simulink model "State_Machine"  (R2024a)
settings: Solver=FixedStepDiscrete  StartTime=0.0  StopTime=10000  RelTol=1e-3
PreLoadFcn:
  | clearEnums;
model workspace (MAT data in the model file):
  Active_Scenario_Index = 1
  BattTempInit = 25
  Battery.SOC_LUT = [0.01 0.02 0.03 0.04 0.05 0.06 0.07 0.08 0.09 0.1 0.11 0.12 0.13 0.14 0.15 0.16 0.17 0.18 0.19 0.2 0.21 0.22 0.23 0.24 0.25 0.26 0.27 0.28 0.29 0.3 0.31 0.32 0.33 0.34 0.35 0.36 0.37 0.38 0.39 0.4 0.41 0.42 0.43 0.44 0.45 0.46 0.47 0.48 0.49 0.5 0.51 0.52 0.53 0.54 0.55 0.56 0.57 0.58 0.59 0.6 0.61 0.62 0.63 0.64 0.65 0.66 0.67 0.68 0.69 0.7 0.71 0.72 0.73 0.74 0.75 0.76 0.77 0.78 0.79 0.8 0.81 0.82 0.83 0.84 0.85 0.86 0.87 0.88 0.89 0.9 0.91 0.92 0.93 0.94 0.95 0.96 0.97 0.98 0.99 1]
  Battery.Temperature_LUT = [-10 0 25 40]
  Battery.Capacity_LUT = [4.04528301887 4.19622641509 4.8 4.73962264151]
  Battery.Em_LUT = [2.67308083891 2.74411674384 2.80408613071 2.86247711994 2.90851059763 2.94904306488 2.9829846776 3.01467102589 3.04031502638 3.06256828113 3.08180972392 3.09994219643 ... (400 elements, 100x4)]
  Battery.R0_LUT = [0.0569026752707 0.0575506938969 0.0576730924021 0.0575627404981 0.0573787336615 0.0571931123197 0.0568199985482 0.056411926464 0.0561974340667 0.0560805640861 0.0557640899305 0.055275807865 ... (400 elements, 100x4)]
  Battery.R1_LUT = [0.0035 0.0035 0.0035 0.0035 0.0035 0.0035 0.0035 0.0035 0.0035 0.0035 0.0035 0.0035 ... (400 elements, 100x4)]
  Battery.C1_LUT = [5000 5000 5000 5000 5000 5000 5000 5000 5000 5000 5000 5000 ... (400 elements, 100x4)]
  Battery.Mass = 0.047
  Battery.ThermalMass = 44
  Battery.R_bleed = 20
  Battery.h_conv = 5
  Battery.cell_area = 0.0037
  Battery.TempInit = 25
  Battery.SOCInit = 0.75
  Battery.Model = 'panasonic ncr18650bd'
  Battery.DischargeCycle_LUT = [1 5 9 13 17 21 25 29 33 37 41 45 49 53 57 61 65 69 73 77 81 85 89 93 97 101 105 109 113 117 121 125 129 133 137 141 145 149 153 157 161 165 169 173 177 181 185 189 193 197 201 205 209 213 217 221 225 229 233 237 241 245 249 253 257 261 265 269 273 277 281 285 289 293 297 301 305 309 313 317]
  Battery.deltaEm_LUT = [0 -0.363115641304 -0.600096647258 -0.689070000839 -0.76773380251 -0.846397604181 -0.926368385458 -0.992711297521 -1.05704974111 -1.12227693902 -1.19018070587 -1.25808447272 -1.31699459748 -1.35876443799 -1.40168267642 -1.44460091485 -1.48751915327 -1.5304373917 -1.57335563013 -1.62198241593 -1.67232184498 -1.71858340023 -1.76179802551 -1.8050126508 -1.84822727608 -1.8917937136 -1.93575272784 -1.97971174208 -2.02367075632 -2.06762977056 -2.11171979109 -2.15588700406 -2.19980020032 -2.24365853098 -2.28751686164 -2.33137519231 -2.37523352297 -2.41909185363 -2.45982559031 -2.49599372373 -2.53216185715 -2.56832999058 -2.604498124 -2.64066625743 -2.67683439085 -2.71300252428 -2.7491706577 -2.78367585394 -2.81632179346 -2.8483348579 -2.88034792233 -2.91236098677 -2.94437405121 -2.97638711564 -3.00840018008 -3.04041324451 -3.07260346059 -3.10359008254 -3.13082308991 -3.15805609728 -3.18528910464 -3.21252211201 -3.23975511938 -3.26698812675 -3.29422113412 -3.32122400938 -3.3463475604 -3.37152613073 -3.39670470105 -3.42188327138 -3.4470618417 -3.47224041203 -3.49938358795 -3.52900276724 -3.55862194653 -3.58824112582 -3.6178603051 -3.64748858268 -3.67711690909 -3.70674523549]
  Battery.deltaCapacity_LUT = [0 -0.860019120059 -1.71332421702 -2.0819400264 -2.45055583577 -2.81917164515 -3.18778745452 -3.48884924257 -3.7808148236 -4.07278040463 -4.36474598566 -4.6567115667 -4.91000721732 -5.08494410056 -5.2598809838 -5.43481786703 -5.60975475027 -5.78469163351 -5.95962851674 -6.13456539998 -6.30950228322 -6.47026795816 -6.62044510558 -6.77062225299 -6.92079940041 -7.07097654783 -7.22115369524 -7.37133084266 -7.52150799007 -7.67168513749 -7.82230984162 -7.97319825819 -8.12408667477 -8.27497509134 -8.42586350792 -8.57675192449 -8.72764034107 -8.87852875764 -9.01789522921 -9.13717923376 -9.25646323831 -9.37574724285 -9.4950312474 -9.61431525195 -9.73359925649 -9.85288326104 -9.97216726558 -10.0914512701 -10.2059878191 -10.3183039593 -10.4306200996 -10.5429362398 -10.65525238 -10.7675685203 -10.8798846605 -10.9922008008 -11.104516941 -11.2125891929 -11.3075699376 -11.4025506823 -11.4975314271 -11.5925121718 -11.6874929166 -11.7824736613 -11.877454406 -11.9716325175 -12.0588579537 -12.1460833899 -12.2333088261 -12.3205342623 -12.4077596986 -12.4949851348 -12.5890165008 -12.6916254178 -12.7942343349 -12.8968432519 -12.999452169 -13.102061086 -13.2046700031 -13.3072789201]
  Battery.cond_thickness = 0.001
  Battery.thermal_conductivity = 205
  CV_Gain = 0.20000000298
  CellType = 1
  HighTempDchrgCurrentLim = Simulink.Signal
  HighTempDchrgCurrentLim.DataType = 'single'
  HighTempDchrgCurrentLim.Dimensions = -1
  HighTempDchrgCurrentLim.DimensionsMode = 'auto'
  HighTempDchrgCurrentLim.Complexity = 'auto'
  HighTempDchrgCurrentLim.SampleTime = -1
  HighTempDchrgCurrentLim.SamplingMode = 'auto'
  HighTempLimit = 50
  I_cc = 30
  LowTempDchrgCurrentLim = Simulink.Signal
  LowTempDchrgCurrentLim.DataType = 'single'
  LowTempDchrgCurrentLim.Dimensions = -1
  LowTempDchrgCurrentLim.DimensionsMode = 'auto'
  LowTempDchrgCurrentLim.Complexity = 'auto'
  LowTempDchrgCurrentLim.SampleTime = -1
  LowTempDchrgCurrentLim.SamplingMode = 'auto'
  LowTempLimit = 5
  MaxCellVoltThrsld = 4.19999980927
  MaxChrgCurrLim = Simulink.Parameter
  MaxChrgCurrLim.Value = 6.36000013351
  MaxChrgCurrLim.Complexity = 'real'
  MaxChrgCurrLim.Dimensions = [1 1]
  MaxChrgCurrLim.DataType = 'single'
  MaxDchrgCurrLim = Simulink.Parameter
  MaxDchrgCurrLim.Value = -20
  MaxDchrgCurrLim.Complexity = 'real'
  MaxDchrgCurrLim.Dimensions = [1 1]
  MaxDchrgCurrLim.DataType = 'single'
  MinCellVoltDchrgCurrentLim = Simulink.Signal
  MinCellVoltDchrgCurrentLim.DataType = 'single'
  MinCellVoltDchrgCurrentLim.Dimensions = -1
  MinCellVoltDchrgCurrentLim.DimensionsMode = 'auto'
  MinCellVoltDchrgCurrentLim.Complexity = 'auto'
  MinCellVoltDchrgCurrentLim.SampleTime = -1
  MinCellVoltDchrgCurrentLim.SamplingMode = 'auto'
  MinCellVoltDchrgCurrentLimTable = Simulink.LookupTable
  MinCellVoltDchrgCurrentLimTable.Table = Simulink.lookuptable.Table
  MinCellVoltDchrgCurrentLimTable.Table.Value = [0 0.5 1]
  MinCellVoltDchrgCurrentLimTable.Table.Dimensions = [1 3]
  MinCellVoltDchrgCurrentLimTable.Table.DataType = 'single'
  MinCellVoltDchrgCurrentLimTable.Table.FieldName = 'DischargeCurrentRate'
  MinCellVoltDchrgCurrentLimTable.Table.Description = 'Discharge Current Rate Based On Mim Cell Voltage'
  MinCellVoltDchrgCurrentLimTable.Breakpoints = Simulink.lookuptable.Breakpoint
  MinCellVoltDchrgCurrentLimTable.Breakpoints.Value = [2.5; 2.75; 3]
  MinCellVoltDchrgCurrentLimTable.Breakpoints.TunableSizeName = 'N1'
  MinCellVoltDchrgCurrentLimTable.Breakpoints.Dimensions = [3 1]
  MinCellVoltDchrgCurrentLimTable.Breakpoints.DataType = 'single'
  MinCellVoltDchrgCurrentLimTable.Breakpoints.Unit = 'V'
  MinCellVoltDchrgCurrentLimTable.Breakpoints.FieldName = 'MinCellVoltage'
  MinCellVoltDchrgCurrentLimTable.Breakpoints.Description = 'Minimum Cell Voltage'
  MinCellVoltDchrgCurrentLimTable.AllowMultipleInstancesOfTypeToHaveDifferentTableBreakpointSizes = 0
  MinCellVoltDchrgCurrentLimTable.SupportTunableSize = 0
  MinCellVoltDchrgCurrentLimTable.StructTypeInfo = Simulink.lookuptable.StructTypeInfo
  MinCellVoltDchrgCurrentLimTable.StructTypeInfo.Name = 'MinCellVoltDchrgCurrentLimTable'
  MinCellVoltDchrgCurrentLimTable.StructTypeInfo.DataScope = 'Auto'
  Np_Module = 31
  Ns_Module = 24
  NumModules = 4
  OverCellVoltageLimit = 4.19999980927
  Sig = Simulink.Signal
  Sig.DataType = 'auto'
  Sig.Dimensions = -1
  Sig.DimensionsMode = 'auto'
  Sig.Complexity = 'auto'
  Sig.SampleTime = -1
  Sig.SamplingMode = 'auto'
  SnsrFltThld = 0.252
  TestCase = 1
  UnderCellVoltageLimit = 2.5
  contactorTime = 200
  currentFactor = 10
  noCurrent = 0
  timeoutContactor = 1
  timeoutCurrent = 1
  ts = 0.1
  vRatio = 0.949999988079
  voltThreshold = 4.09999990463
settings Model: DataDictionary=DD_State_Machine.sldd  ModifiedByFormat=The MathWorks, Inc.  ExtModeTrigDuration=5  Creator=The MathWorks, Inc.  LastModifiedBy=The MathWorks, Inc.
settings SolverCC: AlgebraicLoopSolver=TrustRegion  PositivePriorityOrder=on  AutoInsertRateTranBlk=on  MaxZcPerStep=1
settings DataIOCC: ExternalInput=Battery  SaveOutput=off  SaveTime=off  SignalLoggingName=logsOut
settings OptimizationCC: BlockReduction=off  DefaultParameterBehavior=Inlined  UseFloatMulNetSlope=on  DefaultUnderspecifiedDataType=single  OptimizeBlockIOStorage=off  EnhancedBackFolding=on  PassReuseOutputArgsThreshold=0  ZeroExternalMemoryAtStartup=off  ZeroInternalMemoryAtStartup=off  EfficientFloat2IntCast=on  MaxStackSize=64  OptimizeBlockOrder=speed  DifferentSizesBufferReuse=on
settings DebuggingCC: SignalInfNanChecking=error  SaveWithParameterizedLinksMsg=none  CheckExecutionContextPreStartOutputMsg=on  IntegerOverflowMsg=error  ParameterPrecisionLossMsg=none  ParameterTunabilityLossMsg=error  UnconnectedInputMsg=warning  UnconnectedOutputMsg=warning  UnconnectedLineMsg=warning  AssertControl=DisableAll  PregeneratedLibrarySubsystemCodeDiagnostic=none  SFUnexpectedBacktrackingDiag=warning  SFNoUnconditionalDefaultTransitionDiag=warning  SFExecutionAtInitializationDiag=none  ArithmeticOperatorsInVariantConditions=warning
settings HardwareCC: ProdBitPerLong=64  ProdLongLongMode=on  ProdHWDeviceType=Intel->x86-64 (Linux 64)
settings ModelReferenceCC: EnableRefExpFcnMdlSchedulingChecks=on  ModelReferenceNumInstancesAllowed=Single  PropagateSignalLabelsOutOfModel=off
settings SFSimCC: SimUseLocalCustomCode=off  MATLABDynamicMemAlloc=off  CustomCodeUndefinedFunction=UseInterfaceOnly
settings RTWCC: GenerateReport=on  RTWUseLocalCustomCode=off  BuildConfiguration=Faster Runs  TargetLang=C++  GPUComputeCapability=3.5  DLArmComputeVersion=19.05
settings CodeAppCC: ForceParamTrailComments=on  MaxIdLength=51  OperatorAnnotations=on  MangleLength=4
settings GRTTargetCC: TargetLangStandard=C++03 (ISO)  CodeInterfacePackaging=C++ class
settings ConfigComp: CovMetricSettings=dcw  CovSaveCumulativeToWorkspaceVar=on  CovSaveSingleToWorkspaceVar=on  CovExternalEMLEnable=off  CovSFcnEnable=off  DVMode=DesignErrorDetection  DVMaxProcessTime=7000  DVTestSuiteOptimization=Auto  DVDetectDeadLogic=on  DVDetectIntegerOverflow=off  DVRebuildModelRepresentation=Always

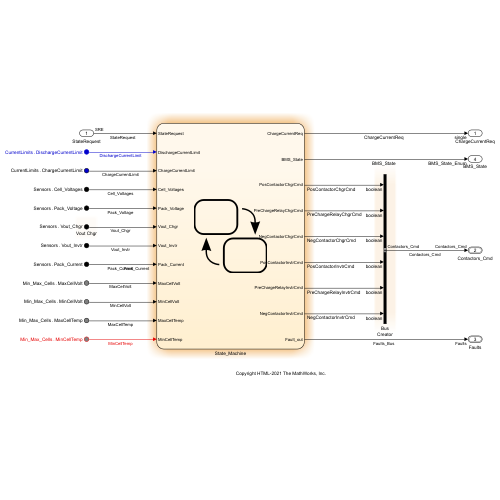
[thumbnail: Simulink's stored preview of the top-level diagram]
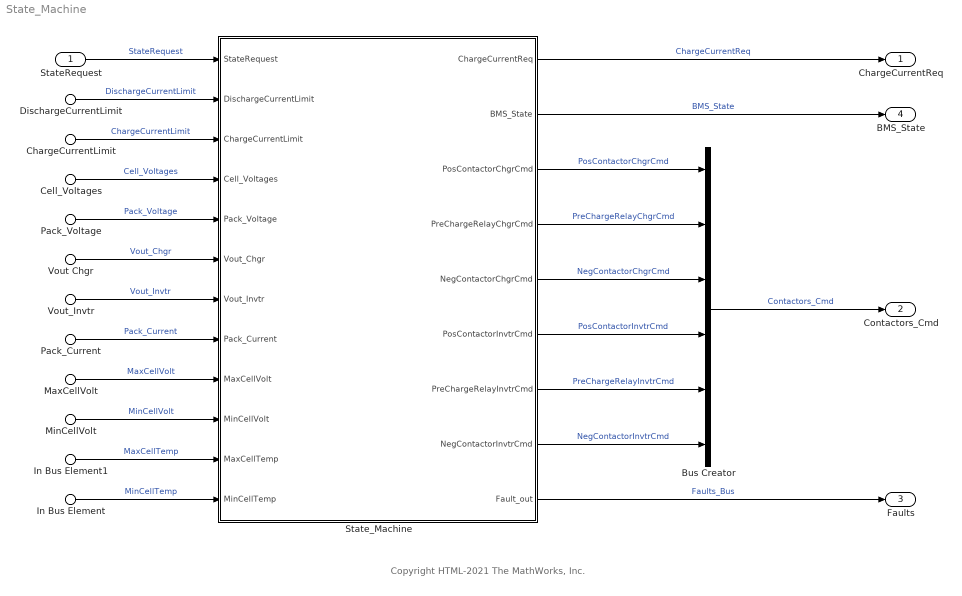
== system State_Machine ==
  note: Copyright HTML-2021 The MathWorks, Inc.
  StateRequest : Inport  OutDataTypeStr=Enum: SRE  PortDimensions=1  SampleTime=[0.10000000000000001,0]
  Cell_Voltages : Inport  Port=2  PortName=Sensors  Element=Cell_Voltages
  Pack_Voltage : Inport  Port=2  PortName=Sensors  Element=Pack_Voltage
  Pack_Current : Inport  Port=2  PortName=Sensors  Element=Pack_Current
  Vout Chgr : Inport  Port=2  PortName=Sensors  Element=Vout_Chgr
  Vout_Invtr : Inport  Port=2  PortName=Sensors  Element=Vout_Invtr
  DischargeCurrentLimit : Inport  Port=3  PortName=CurrentLimits  Element=DischargeCurrentLimit
  ChargeCurrentLimit : Inport  Port=3  PortName=CurrentLimits  Element=ChargeCurrentLimit
  MinCellVolt : Inport  Port=4  PortName=Min_Max_Cells  Element=MinCellVolt
  MaxCellVolt : Inport  Port=4  PortName=Min_Max_Cells  Element=MaxCellVolt
  In Bus Element : Inport  Port=4  PortName=Min_Max_Cells  Element=MinCellTemp
  In Bus Element1 : Inport  Port=4  PortName=Min_Max_Cells  Element=MaxCellTemp
  Bus Creator : BusCreator  Inputs=6  OutDataTypeStr=Bus: Contactors_Cmd  NonVirtualBus=on
      settings: InheritFromInputs=off
  State_Machine : Stateflow chart  TreatAsAtomicUnit=on  VariantControl=(default)
  ChargeCurrentReq : Outport  OutMin=-100  OutMax=100  OutDataTypeStr=single  PortDimensions=1  SampleTime=[0.10000000000000001,0]  VectorParamsAs1DForOutWhenUnconnected=off
  Contactors_Cmd : Outport  Port=2  OutDataTypeStr=Bus: Contactors_Cmd  BusOutputAsStruct=on
  Faults : Outport  Port=3  OutDataTypeStr=Bus: Faults  VectorParamsAs1DForOutWhenUnconnected=off  BusOutputAsStruct=on
  BMS_State : Outport  Port=4  OutDataTypeStr=Enum: BMS_State_Enum  PortDimensions=1  SampleTime=[0.10000000000000001,0]  VectorParamsAs1DForOutWhenUnconnected=off
  wires:
  State_Machine/2(BMS_State) -> BMS_State/1  "BMS_State"
  State_Machine/1(ChargeCurrentReq) -> ChargeCurrentReq/1  "ChargeCurrentReq"
  State_Machine/3(PosContactorChgrCmd) -> Bus Creator/1  "PosContactorChgrCmd"
  State_Machine/4(PreChargeRelayChgrCmd) -> Bus Creator/2  "PreChargeRelayChgrCmd"
  State_Machine/5(NegContactorChgrCmd) -> Bus Creator/3  "NegContactorChgrCmd"
  State_Machine/6(PosContactorInvtrCmd) -> Bus Creator/4  "PosContactorInvtrCmd"
  State_Machine/7(PreChargeRelayInvtrCmd) -> Bus Creator/5  "PreChargeRelayInvtrCmd"
  State_Machine/8(NegContactorInvtrCmd) -> Bus Creator/6  "NegContactorInvtrCmd"
  State_Machine/9(Fault_out) -> Faults/1  "Faults_Bus"
  DischargeCurrentLimit/1 -> State_Machine/2(DischargeCurrentLimit)  "DischargeCurrentLimit"
  ChargeCurrentLimit/1 -> State_Machine/3(ChargeCurrentLimit)  "ChargeCurrentLimit"
  Cell_Voltages/1 -> State_Machine/4(Cell_Voltages)  "Cell_Voltages"
  MinCellVolt/1 -> State_Machine/10(MinCellVolt)  "MinCellVolt"
  MaxCellVolt/1 -> State_Machine/9(MaxCellVolt)  "MaxCellVolt"
  StateRequest/1 -> State_Machine/1(StateRequest)  "StateRequest"
  Pack_Current/1 -> State_Machine/8(Pack_Current)  "Pack_Current"
  Vout_Invtr/1 -> State_Machine/7(Vout_Invtr)  "Vout_Invtr"
  Vout Chgr/1 -> State_Machine/6(Vout_Chgr)  "Vout_Chgr"
  Pack_Voltage/1 -> State_Machine/5(Pack_Voltage)  "Pack_Voltage"
  Bus Creator/1 -> Contactors_Cmd/1  "Contactors_Cmd"
  In Bus Element1/1 -> State_Machine/11(MaxCellTemp)  "MaxCellTemp"
  In Bus Element/1 -> State_Machine/12(MinCellTemp)  "MinCellTemp"

== stateflow chart State_Machine/State_Machine ==
  state Fault Monitoring [group]
    state MonitorCurrLim [parallel]
      settings: executionOrder=1
      state Wait
      state NoCurrLimFault
      state OverCurrentFault
        en:
        FaultPresent = true;
        Fault_out.OverCurrent=true;
      (default) -> NoCurrLimFault : {FaultPresent = false;
          | Fault_out.OverCurrent=false;}
      NoCurrLimFault -> Wait : [(Pack_Current < DischargeCurrentLimit) || ...
          | (Pack_Current > ChargeCurrentLimit)]
      Wait -> NoCurrLimFault [order 2] : [(Pack_Current >= DischargeCurrentLimit) && ...
          | (Pack_Current <= ChargeCurrentLimit)]
      Wait -> OverCurrentFault [order 1] : [after(timeoutCurrent,sec)]
    state MonitorCellVoltage [parallel]
      settings: executionOrder=2
      state OverVoltageFault
        en:
        FaultPresent = true;
        Fault_out.OverVolt = true;
      state NoCellVoltFault
        en,du:
        Delta = abs(Pack_Voltage - sum(Cell_Voltages));
      state SensorFaut
        en:
        FaultPresent = true;
        Fault_out.VoltSensor = true;
      state UnderVoltageFault
        en:
        FaultPresent = true;
        Fault_out.UnderVolt = true;
      (default) -> NoCellVoltFault : {FaultPresent = false;
          | Fault_out.OverVolt = false;
          | Fault_out.UnderVolt = false;
          | Fault_out.VoltSensor = false;
          | }
      NoCellVoltFault -> OverVoltageFault [order 1] : [MaxCellVolt >= ...
          | OverCellVoltageLimit]
      NoCellVoltFault -> SensorFaut [order 2] : [Delta >=...
          |  single(SnsrFltThld)]
      NoCellVoltFault -> UnderVoltageFault [order 3] : [MinCellVolt <=...
          |  UnderCellVoltageLimit]
    state MonitorCellTemp [parallel]
      settings: executionOrder=3
      state HighTemperatureFault
        en:
        FaultPresent = true;
        Fault_out.HighTemp = true;
      state NoCellTempFault
      state LowTemperatureFault
        en:
        FaultPresent = true;
        Fault_out.LowTemp = true;
      (default) -> NoCellTempFault : {FaultPresent = false;
          | Fault_out.HighTemp = false;
          | Fault_out.LowTemp = false;}
      NoCellTempFault -> HighTemperatureFault [order 1] : [MaxCellTemp >= HighTempLimit]
      NoCellTempFault -> LowTemperatureFault [order 2] : [MinCellTemp <= LowTempLimit]
  state MainStateMachine [parallel]
    settings: executionOrder=1
    state Charging
      en:
      BMS_State = BMS_State_Enum.BMS_Charging;
      state Init_Mode
        en:
        ChargeModeReq = Charge_Mode_Enum.Init_Mode;
        ChargeCurrentReq = noCurrent;
      state CC_Mode
        en:
        ChargeModeReq = Charge_Mode_Enum.CC_Mode;
        du:
        ChargeCurrentReq = min(I_cc,ChargeCurrentLimit);
      state CV_Mode
        en:
        ChargeModeReq = Charge_Mode_Enum.CV_Mode;
        du:
        ChargeCurrentReq = ChargeCurrentReq - CV_Gain*(MaxCellVolt - MaxCellVoltThrsld);
        ChargeCurrentReq = min(ChargeCurrentReq, ChargeCurrentLimit);
      (default) -> Init_Mode
      CV_Mode -> Init_Mode : [StateRequest ~= SRE.Charging || ...
          | ChargeCurrentReq <= (I_cc/currentFactor)]
      CC_Mode -> Init_Mode [order 1] : [StateRequest ~= SRE.Charging]
      Init_Mode -> CC_Mode : [StateRequest == SRE.Charging && ...
          | MaxCellVolt < voltThreshold]
      CC_Mode -> CV_Mode [order 2] : [MaxCellVolt>=...
          | MaxCellVoltThrsld]
    state Standby
      en:
      BMS_State = ...
      BMS_State_Enum.BMS_Standby;
    state Driving
      en:
      BMS_State = ...
      BMS_State_Enum.BMS_Driving;
    state Fault
      en,du:
      BMS_State = BMS_State_Enum.BMS_Fault;
    (default) -> Standby
    Standby -> (junction 577) [order 1] : [FaultPresent]
    Standby -> Charging [order 2] : [StateRequest ==SRE.Charging...
        | && ChrgCntctState == Contact.Close]
    (junction 577) -> (junction 580)
    Charging -> Standby [order 3] : [StateRequest ~=SRE.Charging...
        |  && ChrgCntctState == Contact.Init]
    Standby -> Driving [order 3] : [StateRequest == SRE.Driving && ...
        | InvtrCntctState == Contact.Close]
    Driving -> Standby [order 3] : [StateRequest ~= SRE.Driving && ...
        | InvtrCntctState == Contact.Init]
    Driving -> Charging [order 2] : [StateRequest == SRE.Charging && ...
        | ChrgCntctState == Contact.Close]
    Charging -> Driving [order 2] : [StateRequest == SRE.Driving && ...
        | InvtrCntctState == Contact.Close]
    Driving -> Fault [order 1] : [FaultPresent]
    Charging -> Fault [order 1] : [FaultPresent]{ChargeCurrentReq = single(0);}
    (junction 580) -> Fault
  state ChargerContactorState [parallel]
    settings: executionOrder=2
    state OpenChgrContactors
      state ClosePreChrgRly
        PreChargeRelayChgrCmd = true;
      state OpenPosCntct
        PosContactorChgrCmd = false;
      state OpenPreChrgRly
        PreChargeRelayChgrCmd = false;
      state OpenNegCntct
        NegContactorChgrCmd = false;
        ChrgCntctState = Contact.Open;
        PreChrgFault = false;
        Fault_out.Charger = false;
      (default) -> ChargerContactorState.OpenChgrContactors.ClosePreChrgRly : {ChrgCntctState = Contact.Init;}
      ChargerContactorState.OpenChgrContactors.ClosePreChrgRly -> ChargerContactorState.OpenChgrContactors.OpenPosCntct : after(contactorTime,msec) % Check for low current
      ChargerContactorState.OpenChgrContactors.OpenPosCntct -> ChargerContactorState.OpenChgrContactors.OpenPreChrgRly : after(contactorTime,msec)
      ChargerContactorState.OpenChgrContactors.OpenPreChrgRly -> ChargerContactorState.OpenChgrContactors.OpenNegCntct : after(contactorTime,msec)
    state CloseChgrContactors
      state CloseNegCntct
        NegContactorChgrCmd = true;
      state ClosePreChrgRly
        PreChargeRelayChgrCmd = true;
      state ClosePosCntct
        PosContactorChgrCmd = true;
      state OpenPreChrgRly
        PreChargeRelayChgrCmd = false;
        ChrgCntctState = Contact.Close;
      state PreChrgFlt
        PreChrgFault = true;
        Fault_out.Charger = true;
      (default) -> ChargerContactorState.CloseChgrContactors.CloseNegCntct : {ChrgCntctState = Contact.Init;}
      ChargerContactorState.CloseChgrContactors.CloseNegCntct -> ChargerContactorState.CloseChgrContactors.ClosePreChrgRly : after(contactorTime,msec)
      ChargerContactorState.CloseChgrContactors.ClosePreChrgRly -> (junction 564) [order 2]
      (junction 564) -> (junction 566) : after(timeoutContactor,sec)
          | % Check timeout
      ChargerContactorState.CloseChgrContactors.ClosePreChrgRly -> ChargerContactorState.CloseChgrContactors.ClosePosCntct [order 1] : [Vout_Chgr/Pack_Voltage >=vRatio]
      ChargerContactorState.CloseChgrContactors.ClosePosCntct -> ChargerContactorState.CloseChgrContactors.OpenPreChrgRly : after(contactorTime,msec)
      (junction 566) -> ChargerContactorState.CloseChgrContactors.PreChrgFlt
    (default) -> OpenChgrContactors : {ChrgCntctState = Contact.Init;
        | PreChrgFault = false;
        | Fault_out.Charger = false;}
    CloseChgrContactors -> OpenChgrContactors : [StateRequest ~= SRE.Charging || ...
        | FaultPresent]
    OpenChgrContactors -> CloseChgrContactors : [StateRequest == SRE.Charging && ...
        | InvtrCntctState == Contact.Open && ...
        | ~FaultPresent]
  state InverterContactorState [parallel]
    settings: executionOrder=3
    state CloseInvtrContactors
      state CloseNegCntct
        NegContactorInvtrCmd = true;
      state ClosePreChrgRly
        PreChargeRelayInvtrCmd = true;
      state ClosePosCntct
        PosContactorInvtrCmd = true;
      state OpenPreChrgRly
        PreChargeRelayInvtrCmd = false;
        InvtrCntctState = Contact.Close;
      state PreChrgFlt
        PreChrgFault = true;
        Fault_out.Inverter = true;
      (default) -> InverterContactorState.CloseInvtrContactors.CloseNegCntct : {InvtrCntctState = Contact.Init;}
      InverterContactorState.CloseInvtrContactors.CloseNegCntct -> InverterContactorState.CloseInvtrContactors.ClosePreChrgRly : after(contactorTime,msec)
      InverterContactorState.CloseInvtrContactors.ClosePreChrgRly -> (junction 569) [order 2]
      (junction 569) -> (junction 570) : after(timeoutContactor,sec)
          | % Check timeout
      InverterContactorState.CloseInvtrContactors.ClosePreChrgRly -> InverterContactorState.CloseInvtrContactors.ClosePosCntct [order 1] : [Vout_Invtr/Pack_Voltage >=vRatio]
      InverterContactorState.CloseInvtrContactors.ClosePosCntct -> InverterContactorState.CloseInvtrContactors.OpenPreChrgRly : after(contactorTime,msec)
      (junction 570) -> InverterContactorState.CloseInvtrContactors.PreChrgFlt
    state OpenInvtrContactors
      state ClosePreChrgRly
        PreChargeRelayInvtrCmd = true;
      state OpenPosCntct
        PosContactorInvtrCmd = false;
      state OpenPreChrgRly
        PreChargeRelayInvtrCmd = false;
      state OpenNegCntct
        NegContactorInvtrCmd = false;
        InvtrCntctState = Contact.Open;
        PreChrgFault = false;
        Fault_out.Inverter = false;
      (default) -> InverterContactorState.OpenInvtrContactors.ClosePreChrgRly : {InvtrCntctState = Contact.Init;}
      InverterContactorState.OpenInvtrContactors.ClosePreChrgRly -> InverterContactorState.OpenInvtrContactors.OpenPosCntct : after(contactorTime,msec) % Check for low current
      InverterContactorState.OpenInvtrContactors.OpenPosCntct -> InverterContactorState.OpenInvtrContactors.OpenPreChrgRly : after(contactorTime,msec)
      InverterContactorState.OpenInvtrContactors.OpenPreChrgRly -> InverterContactorState.OpenInvtrContactors.OpenNegCntct : after(contactorTime,msec)
    (default) -> OpenInvtrContactors : {InvtrCntctState =Contact.Init;
        | PreChrgFault = false;
        | Fault_out.Inverter = false;}
    CloseInvtrContactors -> OpenInvtrContactors : [StateRequest ~= SRE.Driving || ...
        | FaultPresent]
    OpenInvtrContactors -> CloseInvtrContactors : [StateRequest == SRE.Driving && ...
        | ChrgCntctState == Contact.Open && ...
        | ~FaultPresent]
  data: StateRequest input Enum: SRE; DischargeCurrentLimit input single; ChargeCurrentLimit input single; Cell_Voltages input single; Pack_Voltage input single; Vout_Chgr input single; Vout_Invtr input single; Pack_Current input single; ChargeCurrentReq output; I_cc parameter; MaxCellVolt input single; BMS_State output Enum: BMS_State_Enum =BMS_State_Enum.BMS_Standby; PosContactorChgrCmd output boolean; PreChargeRelayChgrCmd output; NegContactorChgrCmd output; PosContactorInvtrCmd output; PreChargeRelayInvtrCmd output; NegContactorInvtrCmd output; ChrgCntctState local Enum: Contact; InvtrCntctState local Enum: Contact; PreChrgFault local; MaxCellVoltThrsld parameter; FaultPresent local; MinCellVolt input single; OverCellVoltageLimit parameter; UnderCellVoltageLimit parameter; Delta local; HighTempLimit parameter; LowTempLimit parameter; SnsrFltThld parameter; CV_Gain parameter; ChargeModeReq local Enum: Charge_Mode_Enum =Charge_Mode_Enum.Init_Mode; MonitorCurrLimMode local Enum: MonitorCurrLimModeType; MonitorCellVoltageMode local Enum: MonitorCellVoltageModeType; MonitorCellTempMode local Enum: MonitorCellTempModeType; Fault_out output Bus: Faults; contactorTime parameter uint16; timeoutContactor parameter uint8; timeoutCurrent parameter uint8; vRatio parameter single; voltThreshold parameter single; currentFactor parameter single; noCurrent parameter single; MaxCellTemp input; MinCellTemp input
